simulink model "accAndGyroFiltered"  (R2016b)
settings: Solver=VariableStepAuto  StartTime=0.0  StopTime=50  RelTol=1e-3
undefined symbols (not defined in the file): DiscIntNeverNeededParam
libraries: simulink_extras x5, dspfdesign x1
settings Model: Creator=vibek  LastModifiedBy=vibek

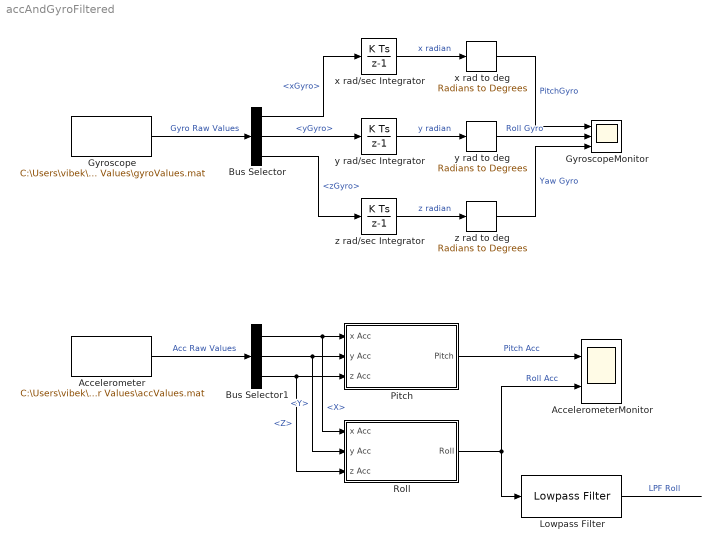
== system accAndGyroFiltered ==
  Accelerometer : FromFile  FileName=C:\Users\vibek\Documents\MATLAB\Simulink\Projects\models\Sensor Values\accValues.mat  OutDataTypeStr=Bus: accResult  SampleTime=0.01
  AccelerometerMonitor : Scope  NumInputPorts=2
  Bus Selector : BusSelector  OutputSignals=xGyro,yGyro,zGyro
  Bus Selector1 : BusSelector  OutputSignals=X,Y,Z
  Gyroscope : FromFile  FileName=C:\Users\vibek\Documents\MATLAB\Simulink\Projects\models\Sensor Values\gyroValues.mat  OutDataTypeStr=Bus: gyroResult  SampleTime=0.01
  GyroscopeMonitor : Scope  NumInputPorts=3
  Lowpass Filter : dspfdesign/Lowpass Filter  FilterType=FIR  DesignForMinimumOrder=on  FilterOrder=50  PassbandFrequency=7  StopbandFrequency=8  PassbandRipple=1  StopbandAttenuation=10  InheritSampleRate=on  SampleRate=100  SimulateUsing=Interpreted execution  roundingMode=Floor  coeffsDataTypeStr=fixdt(1,16)
  Pitch : Subsystem
  Roll : Subsystem
  x rad to deg : simulink_extras/Transformations/Radians to Degrees
  x rad/sec Integrator : DiscreteIntegrator  gainval=1  InitialConditionSetting=State (most efficient)  SampleTime=0.01  ICPrevOutput=DiscIntNeverNeededParam  ICPrevScaledInput=DiscIntNeverNeededParam
  y rad to deg : simulink_extras/Transformations/Radians to Degrees
  y rad/sec Integrator : DiscreteIntegrator  gainval=1  InitialConditionSetting=State (most efficient)  SampleTime=-1  ICPrevOutput=DiscIntNeverNeededParam  ICPrevScaledInput=DiscIntNeverNeededParam
  z rad to deg : simulink_extras/Transformations/Radians to Degrees
  z rad/sec Integrator : DiscreteIntegrator  gainval=1  InitialConditionSetting=State (most efficient)  SampleTime=-1  ICPrevOutput=DiscIntNeverNeededParam  ICPrevScaledInput=DiscIntNeverNeededParam
  wires:
  Gyroscope/1 -> Bus Selector/1  "Gyro Raw Values"
  Bus Selector/1 -> x rad/sec Integrator/1  "<xGyro>"
  Bus Selector/2 -> y rad/sec Integrator/1  "<yGyro>"
  x rad/sec Integrator/1 -> x rad to deg/1  "x radian"
  y rad/sec Integrator/1 -> y rad to deg/1  "y radian"
  z rad/sec Integrator/1 -> z rad to deg/1  "z radian"
  Bus Selector/3 -> z rad/sec Integrator/1  "<zGyro>"
  y rad to deg/1 -> GyroscopeMonitor/2  "Roll Gyro"
  x rad to deg/1 -> GyroscopeMonitor/1  "PitchGyro"
  z rad to deg/1 -> GyroscopeMonitor/3  "Yaw Gyro"
  Accelerometer/1 -> Bus Selector1/1  "Acc Raw Values"
  Bus Selector1/1 -> Roll/1(x Acc), Pitch/1(x Acc)  "<X>"
  Bus Selector1/2 -> Roll/2(y Acc), Pitch/2(y Acc)  "<Y>"
  Bus Selector1/3 -> Roll/3(z Acc), Pitch/3(z Acc)  "<Z>"
  Pitch/1(Pitch) -> AccelerometerMonitor/1  "Pitch Acc"
  Roll/1(Roll) -> Lowpass Filter/1, AccelerometerMonitor/2  "Roll Acc"
  Lowpass Filter/1 -> ?  "LPF Roll"

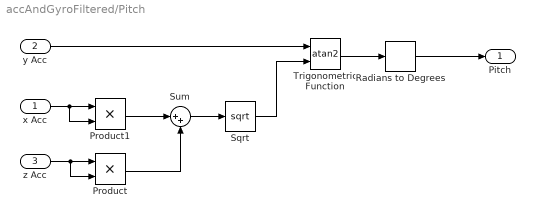
== system accAndGyroFiltered/Pitch ==
  x Acc : Inport
  y Acc : Inport  Port=2
  z Acc : Inport  Port=3
  Product : Product
  Product1 : Product
  Radians to Degrees : simulink_extras/Transformations/Radians to Degrees
  Sqrt : Sqrt  SaturateOnIntegerOverflow=on
  Sum : Sum  Inputs=|++
  Trigonometric Function : Trigonometry  Operator=atan2
  Pitch : Outport
  wires:
  Radians to Degrees/1 -> Pitch/1
  Trigonometric Function/1 -> Radians to Degrees/1
  Sqrt/1 -> Trigonometric Function/2
  Sum/1 -> Sqrt/1
  Product/1 -> Sum/2
  Product1/1 -> Sum/1
  z Acc/1 -> Product/1, Product/2
  x Acc/1 -> Product1/2, Product1/1
  y Acc/1 -> Trigonometric Function/1

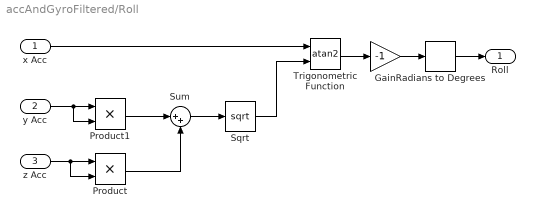
== system accAndGyroFiltered/Roll ==
  x Acc : Inport
  y Acc : Inport  Port=2
  z Acc : Inport  Port=3
  Gain : Gain  Gain=-1
  Product : Product
  Product1 : Product
  Radians to Degrees : simulink_extras/Transformations/Radians to Degrees
  Sqrt : Sqrt  SaturateOnIntegerOverflow=on
  Sum : Sum  Inputs=|++
  Trigonometric Function : Trigonometry  Operator=atan2
  Roll : Outport
  wires:
  z Acc/1 -> Product/2, Product/1
  y Acc/1 -> Product1/2, Product1/1
  Product1/1 -> Sum/1
  Product/1 -> Sum/2
  Sum/1 -> Sqrt/1
  x Acc/1 -> Trigonometric Function/1
  Sqrt/1 -> Trigonometric Function/2
  Trigonometric Function/1 -> Gain/1
  Radians to Degrees/1 -> Roll/1
  Gain/1 -> Radians to Degrees/1
